simulink model "model_QK_SFSVD_ROS"  (Simulink 7.6)
settings: Solver=FixedStepDiscrete  SolverMode=SingleTasking  StartTime=0  StopTime=100  FixedStep=0.01  RelTol=1e-3
values from neighbouring files (symbols this model uses):
  parameter = block.DialogPrm(3).Data    [Kalmangain.m]    (also in init_QK_ROS.m = load('parameter'); statePrediction.m = block.DialogPrm(2).Data)
libraries: PortLib x11, simulink x2, aerolibutil x2
(part 3 of 4)

== matlab function Kalmanfilter/statePrediction ==
  data: uin input double; x_pred output double; xin input double; dt input double; parameter parameter double
function x_pred = statePrediction(uin, xin, dt, parameter)

% parameters
g       = parameter.g;  
m       = parameter.m;
l_m     = parameter.l_m; 
I_x     = parameter.I_x;
I_y     = parameter.I_y;
I_z     = parameter.I_z; 
Psi     = parameter.Psi; 
R_A     = parameter.R_A;
J_M     = parameter.J_M;
CT2s    = parameter.CT2s;
CT1s    = parameter.CT1s;
C_wz    = parameter.C_wz;
C_mxy   = parameter.C_mxy;
C_mz    = parameter.C_mz;
alpha_m = parameter.alpha_m;
beta_m  = parameter.beta_m;
k_m     = parameter.k_m;

% input vector
U_1 = uin(1);
U_2 = uin(2);
U_3 = uin(3);
U_4 = uin(4);

% old state vector
% p_x = xin(1);
% p_y = xin(2);
% p_z = xin(3);
u = xin(4);
v = xin(5);
w = xin(6);
q_0 = xin(7);
q_1 = xin(8);
q_2 = xin(9);
q_3 = xin(10);
% a_x_bias = xin(11);
% a_y_bias = xin(12);
% a_z_bias = xin(13);
% p_bias = xin(14);
% q_bias = xin(15);
% r_bias = xin(16);
p = xin(17);
q = xin(18);
r = xin(19);
w_1 = xin(20);
w_2 = xin(21);
w_3 = xin(22);
w_4 = xin(23);
k_t = xin(24);
CT0s = xin(25);
M_x0 = xin(26);
M_y0 = xin(27);
M_z0 = xin(28);
v_x_wind = xin(29);
v_y_wind = xin(30);
C_wxy = xin(31);

vx_res = -u+v_x_wind*(q_0*q_0+q_1*q_1-q_2*q_2-q_3*q_3)+v_y_wind*(q_0*q_3*2.0+q_1*q_2*2.0);
vy_res = v-v_y_wind*(q_0*q_0-q_1*q_1+q_2*q_2-q_3*q_3)+v_x_wind*(q_0*q_3*2.0-q_1*q_2*2.0);
vz_res = w-v_x_wind*(q_0*q_2*2.0+q_1*q_3*2.0)+v_y_wind*(q_0*q_1*2.0-q_2*q_3*2.0);
velocityLength = sqrt(eps + vx_res^2 + vy_res^2 + vz_res^2);

dx = zeros(31,1);
if min(uin) > 3
    dx(1) = u*(q_0*q_0+q_1*q_1-q_2*q_2-q_3*q_3)-v*(q_0*q_3*2.0-q_1*q_2*2.0)+w*(q_0*q_2*2.0+q_1*q_3*2.0);
    dx(2) = v*(q_0*q_0-q_1*q_1+q_2*q_2-q_3*q_3)+u*(q_0*q_3*2.0+q_1*q_2*2.0)-w*(q_0*q_1*2.0-q_2*q_3*2.0);
    dx(3) = w*(q_0*q_0-q_1*q_1-q_2*q_2+q_3*q_3)-u*(q_0*q_2*2.0-q_1*q_3*2.0)+v*(q_0*q_1*2.0+q_2*q_3*2.0);
    dx(4) = -q*w+r*v-g*(q_0*q_2*2.0-q_1*q_3*2.0)+(C_wxy*(vx_res)*velocityLength)/m;
    dx(5) = p*w-r*u+g*(q_0*q_1*2.0+q_2*q_3*2.0)-(C_wxy*velocityLength*(vy_res))/m;
    dx(6) = g*(q_0*q_0-q_1*q_1-q_2*q_2+q_3*q_3)-p*v+q*u-(CT0s*(w_1*w_1)+CT0s*(w_2*w_2)+CT0s*(w_3*w_3)+CT0s*(w_4*w_4)-CT1s*w_2*(w+l_m*p+q_0*q_1*v_y_wind*2.0-q_0*q_2*v_x_wind*2.0-q_1*q_3*v_x_wind*2.0-q_2*q_3*v_y_wind*2.0)-CT1s*w_3*(w+l_m*q+q_0*q_1*v_y_wind*2.0-q_0*q_2*v_x_wind*2.0-q_1*q_3*v_x_wind*2.0-q_2*q_3*v_y_wind*2.0)+CT1s*w_4*(-w+l_m*p-q_0*q_1*v_y_wind*2.0+q_0*q_2*v_x_wind*2.0+q_1*q_3*v_x_wind*2.0+q_2*q_3*v_y_wind*2.0)+CT1s*w_1*(-w+l_m*q-q_0*q_1*v_y_wind*2.0+q_0*q_2*v_x_wind*2.0+q_1*q_3*v_x_wind*2.0+q_2*q_3*v_y_wind*2.0)+CT2s*abs(-w+l_m*p-q_0*q_1*v_y_wind*2.0+q_0*q_2*v_x_wind*2.0+q_1*q_3*v_x_wind*2.0+q_2*q_3*v_y_wind*2.0)*(-w+l_m*p-q_0*q_1*v_y_wind*2.0+q_0*q_2*v_x_wind*2.0+q_1*q_3*v_x_wind*2.0+q_2*q_3*v_y_wind*2.0)+CT2s*abs(-w+l_m*q-q_0*q_1*v_y_wind*2.0+q_0*q_2*v_x_wind*2.0+q_1*q_3*v_x_wind*2.0+q_2*q_3*v_y_wind*2.0)*(-w+l_m*q-q_0*q_1*v_y_wind*2.0+q_0*q_2*v_x_wind*2.0+q_1*q_3*v_x_wind*2.0+q_2*q_3*v_y_wind*2.0)-CT2s*abs(w+l_m*p+q_0*q_1*v_y_wind*2.0-q_0*q_2*v_x_wind*2.0-q_1*q_3*v_x_wind*2.0-q_2*q_3*v_y_wind*2.0)*(w+l_m*p+q_0*q_1*v_y_wind*2.0-q_0*q_2*v_x_wind*2.0-q_1*q_3*v_x_wind*2.0-q_2*q_3*v_y_wind*2.0)-CT2s*abs(w+l_m*q+q_0*q_1*v_y_wind*2.0-q_0*q_2*v_x_wind*2.0-q_1*q_3*v_x_wind*2.0-q_2*q_3*v_y_wind*2.0)*(w+l_m*q+q_0*q_1*v_y_wind*2.0-q_0*q_2*v_x_wind*2.0-q_1*q_3*v_x_wind*2.0-q_2*q_3*v_y_wind*2.0))/m-(C_wz*(vz_res)*velocityLength)/m;
    dx(7) = p*q_1*(-1.0/2.0)-q*q_2*(1.0/2.0)-q_3*r*(1.0/2.0)-q_0*((q_0*q_0)*3.0+(q_1*q_1)*3.0+(q_2*q_2)*3.0+(q_3*q_3)*3.0-3.0);
    dx(8) = p*q_0*(1.0/2.0)-q*q_3*(1.0/2.0)+q_2*r*(1.0/2.0)-q_1*((q_0*q_0)*3.0+(q_1*q_1)*3.0+(q_2*q_2)*3.0+(q_3*q_3)*3.0-3.0);
    dx(9) = p*q_3*(1.0/2.0)+q*q_0*(1.0/2.0)-q_1*r*(1.0/2.0)-q_2*((q_0*q_0)*3.0+(q_1*q_1)*3.0+(q_2*q_2)*3.0+(q_3*q_3)*3.0-3.0);
    dx(10) = p*q_2*(-1.0/2.0)+q*q_1*(1.0/2.0)+q_0*r*(1.0/2.0)-q_3*((q_0*q_0)*3.0+(q_1*q_1)*3.0+(q_2*q_2)*3.0+(q_3*q_3)*3.0-3.0);
    dx(17) = (M_x0-C_mxy*p*sqrt(p*p+q*q+r*r)+I_y*q*r-I_z*q*r-CT0s*l_m*(w_2*w_2)+CT0s*l_m*(w_4*w_4)+CT2s*(l_m*l_m)*p*abs(w+l_m*p+q_0*q_1*v_y_wind*2.0-q_0*q_2*v_x_wind*2.0-q_1*q_3*v_x_wind*2.0-q_2*q_3*v_y_wind*2.0)-CT2s*l_m*w*abs(-w+l_m*p-q_0*q_1*v_y_wind*2.0+q_0*q_2*v_x_wind*2.0+q_1*q_3*v_x_wind*2.0+q_2*q_3*v_y_wind*2.0)+CT1s*(l_m*l_m)*p*w_2+CT1s*(l_m*l_m)*p*w_4+CT2s*(l_m*l_m)*p*abs(-w+l_m*p-q_0*q_1*v_y_wind*2.0+q_0*q_2*v_x_wind*2.0+q_1*q_3*v_x_wind*2.0+q_2*q_3*v_y_wind*2.0)+CT2s*l_m*w*abs(w+l_m*p+q_0*q_1*v_y_wind*2.0-q_0*q_2*v_x_wind*2.0-q_1*q_3*v_x_wind*2.0-q_2*q_3*v_y_wind*2.0)+CT1s*l_m*w*w_2-CT1s*l_m*w*w_4-CT2s*l_m*q_0*q_1*v_y_wind*abs(-w+l_m*p-q_0*q_1*v_y_wind*2.0+q_0*q_2*v_x_wind*2.0+q_1*q_3*v_x_wind*2.0+q_2*q_3*v_y_wind*2.0)*2.0+CT2s*l_m*q_0*q_2*v_x_wind*abs(-w+l_m*p-q_0*q_1*v_y_wind*2.0+q_0*q_2*v_x_wind*2.0+q_1*q_3*v_x_wind*2.0+q_2*q_3*v_y_wind*2.0)*2.0+CT2s*l_m*q_1*q_3*v_x_wind*abs(-w+l_m*p-q_0*q_1*v_y_wind*2.0+q_0*q_2*v_x_wind*2.0+q_1*q_3*v_x_wind*2.0+q_2*q_3*v_y_wind*2.0)*2.0+CT2s*l_m*q_2*q_3*v_y_wind*abs(-w+l_m*p-q_0*q_1*v_y_wind*2.0+q_0*q_2*v_x_wind*2.0+q_1*q_3*v_x_wind*2.0+q_2*q_3*v_y_wind*2.0)*2.0+CT2s*l_m*q_0*q_1*v_y_wind*abs(w+l_m*p+q_0*q_1*v_y_wind*2.0-q_0*q_2*v_x_wind*2.0-q_1*q_3*v_x_wind*2.0-q_2*q_3*v_y_wind*2.0)*2.0-CT2s*l_m*q_0*q_2*v_x_wind*abs(w+l_m*p+q_0*q_1*v_y_wind*2.0-q_0*q_2*v_x_wind*2.0-q_1*q_3*v_x_wind*2.0-q_2*q_3*v_y_wind*2.0)*2.0-CT2s*l_m*q_1*q_3*v_x_wind*abs(w+l_m*p+q_0*q_1*v_y_wind*2.0-q_0*q_2*v_x_wind*2.0-q_1*q_3*v_x_wind*2.0-q_2*q_3*v_y_wind*2.0)*2.0-CT2s*l_m*q_2*q_3*v_y_wind*abs(w+l_m*p+q_0*q_1*v_y_wind*2.0-q_0*q_2*v_x_wind*2.0-q_1*q_3*v_x_wind*2.0-q_2*q_3*v_y_wind*2.0)*2.0+CT1s*l_m*q_0*q_1*v_y_wind*w_2*2.0-CT1s*l_m*q_0*q_2*v_x_wind*w_2*2.0-CT1s*l_m*q_0*q_1*v_y_wind*w_4*2.0+CT1s*l_m*q_0*q_2*v_x_wind*w_4*2.0-CT1s*l_m*q_1*q_3*v_x_wind*w_2*2.0+CT1s*l_m*q_1*q_3*v_x_wind*w_4*2.0-CT1s*l_m*q_2*q_3*v_y_wind*w_2*2.0+CT1s*l_m*q_2*q_3*v_y_wind*w_4*2.0)/I_x;
    dx(18) = (M_y0-C_mxy*q*sqrt(p*p+q*q+r*r)-I_x*p*r+I_z*p*r+CT0s*l_m*(w_1*w_1)-CT0s*l_m*(w_3*w_3)+CT2s*(l_m*l_m)*q*abs(w+l_m*q+q_0*q_1*v_y_wind*2.0-q_0*q_2*v_x_wind*2.0-q_1*q_3*v_x_wind*2.0-q_2*q_3*v_y_wind*2.0)-CT2s*l_m*w*abs(-w+l_m*q-q_0*q_1*v_y_wind*2.0+q_0*q_2*v_x_wind*2.0+q_1*q_3*v_x_wind*2.0+q_2*q_3*v_y_wind*2.0)+CT1s*(l_m*l_m)*q*w_1+CT1s*(l_m*l_m)*q*w_3+CT2s*(l_m*l_m)*q*abs(-w+l_m*q-q_0*q_1*v_y_wind*2.0+q_0*q_2*v_x_wind*2.0+q_1*q_3*v_x_wind*2.0+q_2*q_3*v_y_wind*2.0)+CT2s*l_m*w*abs(w+l_m*q+q_0*q_1*v_y_wind*2.0-q_0*q_2*v_x_wind*2.0-q_1*q_3*v_x_wind*2.0-q_2*q_3*v_y_wind*2.0)-CT1s*l_m*w*w_1+CT1s*l_m*w*w_3-CT2s*l_m*q_0*q_1*v_y_wind*abs(-w+l_m*q-q_0*q_1*v_y_wind*2.0+q_0*q_2*v_x_wind*2.0+q_1*q_3*v_x_wind*2.0+q_2*q_3*v_y_wind*2.0)*2.0+CT2s*l_m*q_0*q_2*v_x_wind*abs(-w+l_m*q-q_0*q_1*v_y_wind*2.0+q_0*q_2*v_x_wind*2.0+q_1*q_3*v_x_wind*2.0+q_2*q_3*v_y_wind*2.0)*2.0+CT2s*l_m*q_1*q_3*v_x_wind*abs(-w+l_m*q-q_0*q_1*v_y_wind*2.0+q_0*q_2*v_x_wind*2.0+q_1*q_3*v_x_wind*2.0+q_2*q_3*v_y_wind*2.0)*2.0+CT2s*l_m*q_2*q_3*v_y_wind*abs(-w+l_m*q-q_0*q_1*v_y_wind*2.0+q_0*q_2*v_x_wind*2.0+q_1*q_3*v_x_wind*2.0+q_2*q_3*v_y_wind*2.0)*2.0+CT2s*l_m*q_0*q_1*v_y_wind*abs(w+l_m*q+q_0*q_1*v_y_wind*2.0-q_0*q_2*v_x_wind*2.0-q_1*q_3*v_x_wind*2.0-q_2*q_3*v_y_wind*2.0)*2.0-CT2s*l_m*q_0*q_2*v_x_wind*abs(w+l_m*q+q_0*q_1*v_y_wind*2.0-q_0*q_2*v_x_wind*2.0-q_1*q_3*v_x_wind*2.0-q_2*q_3*v_y_wind*2.0)*2.0-CT2s*l_m*q_1*q_3*v_x_wind*abs(w+l_m*q+q_0*q_1*v_y_wind*2.0-q_0*q_2*v_x_wind*2.0-q_1*q_3*v_x_wind*2.0-q_2*q_3*v_y_wind*2.0)*2.0-CT2s*l_m*q_2*q_3*v_y_wind*abs(w+l_m*q+q_0*q_1*v_y_wind*2.0-q_0*q_2*v_x_wind*2.0-q_1*q_3*v_x_wind*2.0-q_2*q_3*v_y_wind*2.0)*2.0-CT1s*l_m*q_0*q_1*v_y_wind*w_1*2.0+CT1s*l_m*q_0*q_2*v_x_wind*w_1*2.0+CT1s*l_m*q_0*q_1*v_y_wind*w_3*2.0-CT1s*l_m*q_0*q_2*v_x_wind*w_3*2.0+CT1s*l_m*q_1*q_3*v_x_wind*w_1*2.0-CT1s*l_m*q_1*q_3*v_x_wind*w_3*2.0+CT1s*l_m*q_2*q_3*v_y_wind*w_1*2.0-CT1s*l_m*q_2*q_3*v_y_wind*w_3*2.0)/I_y;
    dx(19) = ((Psi*Psi)*w_1*(1.0/2.0)-(Psi*Psi)*w_2*(1.0/2.0)+(Psi*Psi)*w_3*(1.0/2.0)-(Psi*Psi)*w_4*(1.0/2.0)+M_z0*R_A-Psi*sqrt((U_1*U_1)*(beta_m*beta_m)+(Psi*Psi)*(w_1*w_1)+R_A*U_1*alpha_m*4.0-Psi*U_1*beta_m*w_1*2.0)*(1.0/2.0)+Psi*sqrt((U_2*U_2)*(beta_m*beta_m)+(Psi*Psi)*(w_2*w_2)+R_A*U_2*alpha_m*4.0-Psi*U_2*beta_m*w_2*2.0)*(1.0/2.0)-Psi*sqrt((U_3*U_3)*(beta_m*beta_m)+(Psi*Psi)*(w_3*w_3)+R_A*U_3*alpha_m*4.0-Psi*U_3*beta_m*w_3*2.0)*(1.0/2.0)+Psi*sqrt((U_4*U_4)*(beta_m*beta_m)+(Psi*Psi)*(w_4*w_4)+R_A*U_4*alpha_m*4.0-Psi*U_4*beta_m*w_4*2.0)*(1.0/2.0)-Psi*U_1*beta_m*(1.0/2.0)+Psi*U_2*beta_m*(1.0/2.0)-Psi*U_3*beta_m*(1.0/2.0)+Psi*U_4*beta_m*(1.0/2.0)-C_mz*R_A*r*sqrt(p*p+q*q+r*r)+I_x*R_A*p*q-I_y*R_A*p*q)/(I_z*R_A);
    dx(20) = (-k_m*w_1+Psi*(sqrt(1.0/(R_A*R_A)*power(U_1*beta_m-Psi*w_1,2.0)*(1.0/4.0)+(U_1*alpha_m)/R_A)+(U_1*beta_m*(1.0/2.0)-Psi*w_1*(1.0/2.0))/R_A)+k_t*(-CT0s*(w_1*w_1)+CT2s*abs(w-l_m*q-v_x_wind*(q_0*q_2*2.0+q_1*q_3*2.0)+v_y_wind*(q_0*q_1*2.0-q_2*q_3*2.0))*(w-l_m*q-v_x_wind*(q_0*q_2*2.0+q_1*q_3*2.0)+v_y_wind*(q_0*q_1*2.0-q_2*q_3*2.0))+CT1s*w_1*(w-l_m*q-v_x_wind*(q_0*q_2*2.0+q_1*q_3*2.0)+v_y_wind*(q_0*q_1*2.0-q_2*q_3*2.0))))/J_M;
    dx(21) = (-k_m*w_2+k_t*(-CT0s*(w_2*w_2)+CT2s*abs(w+l_m*p-v_x_wind*(q_0*q_2*2.0+q_1*q_3*2.0)+v_y_wind*(q_0*q_1*2.0-q_2*q_3*2.0))*(w+l_m*p-v_x_wind*(q_0*q_2*2.0+q_1*q_3*2.0)+v_y_wind*(q_0*q_1*2.0-q_2*q_3*2.0))+CT1s*w_2*(w+l_m*p-v_x_wind*(q_0*q_2*2.0+q_1*q_3*2.0)+v_y_wind*(q_0*q_1*2.0-q_2*q_3*2.0)))+Psi*(sqrt(1.0/(R_A*R_A)*power(U_2*beta_m-Psi*w_2,2.0)*(1.0/4.0)+(U_2*alpha_m)/R_A)+(U_2*beta_m*(1.0/2.0)-Psi*w_2*(1.0/2.0))/R_A))/J_M;
    dx(22) = (-k_m*w_3+Psi*(sqrt(1.0/(R_A*R_A)*power(U_3*beta_m-Psi*w_3,2.0)*(1.0/4.0)+(U_3*alpha_m)/R_A)+(U_3*beta_m*(1.0/2.0)-Psi*w_3*(1.0/2.0))/R_A)+k_t*(-CT0s*(w_3*w_3)+CT2s*abs(w+l_m*q-v_x_wind*(q_0*q_2*2.0+q_1*q_3*2.0)+v_y_wind*(q_0*q_1*2.0-q_2*q_3*2.0))*(w+l_m*q-v_x_wind*(q_0*q_2*2.0+q_1*q_3*2.0)+v_y_wind*(q_0*q_1*2.0-q_2*q_3*2.0))+CT1s*w_3*(w+l_m*q-v_x_wind*(q_0*q_2*2.0+q_1*q_3*2.0)+v_y_wind*(q_0*q_1*2.0-q_2*q_3*2.0))))/J_M;
    dx(23) = (-k_m*w_4+k_t*(-CT0s*(w_4*w_4)+CT2s*abs(w-l_m*p-v_x_wind*(q_0*q_2*2.0+q_1*q_3*2.0)+v_y_wind*(q_0*q_1*2.0-q_2*q_3*2.0))*(w-l_m*p-v_x_wind*(q_0*q_2*2.0+q_1*q_3*2.0)+v_y_wind*(q_0*q_1*2.0-q_2*q_3*2.0))+CT1s*w_4*(w-l_m*p-v_x_wind*(q_0*q_2*2.0+q_1*q_3*2.0)+v_y_wind*(q_0*q_1*2.0-q_2*q_3*2.0)))+Psi*(sqrt(1.0/(R_A*R_A)*power(U_4*beta_m-Psi*w_4,2.0)*(1.0/4.0)+(U_4*alpha_m)/R_A)+(U_4*beta_m*(1.0/2.0)-Psi*w_4*(1.0/2.0))/R_A))/J_M;
end

% state prediction

x_pred = xin + dt*dx;
